simulink model "BloquesP1"  (R2024a)
settings: Solver=VariableStepAuto  StartTime=0.0  StopTime=20  MaxStep=0.001  RelTol=1e-5
values from neighbouring files (symbols this model uses):
  Beq = 4.3    [Practica1FunOde.m]
  Bp = 0.0024    [Practica1FunOde.m]
  Fc = 0    [Practica1FunOde.m]
  g = -9.81    [Practica1FunOde.m]
  Ip = 0.0079    [Practica1FunOde.m]
  lp = 0.3302    [Practica1FunOde.m]
  Mc = 0.7031    [Practica1FunOde.m]
  Mp = 0.23    [Practica1FunOde.m]
settings Model: Creator=52331  LastModifiedBy=52331

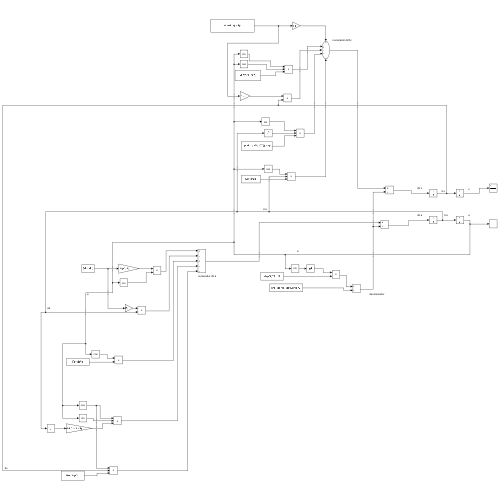
[thumbnail: Simulink's stored preview of the top-level diagram]
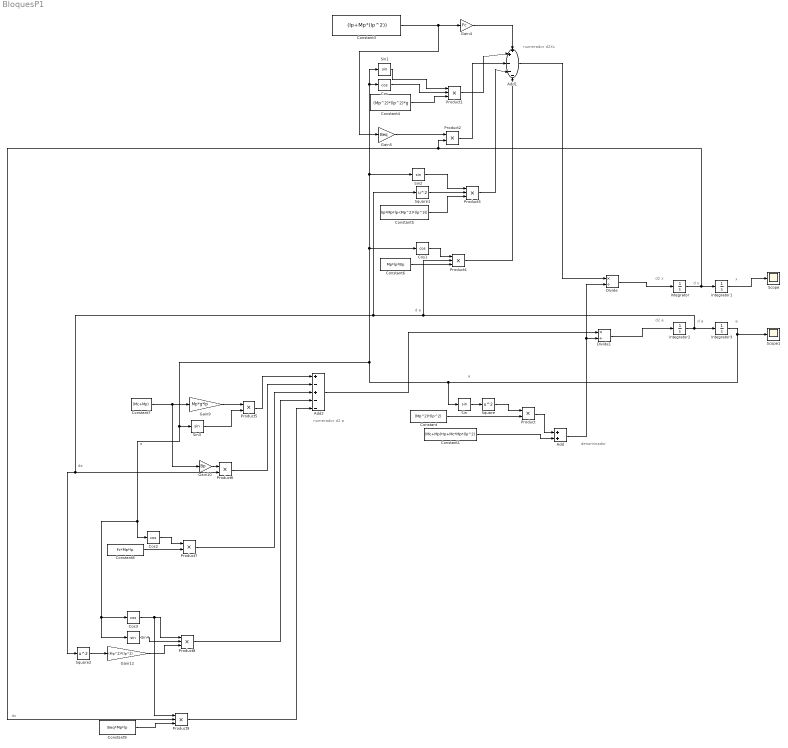
== system BloquesP1 ==
  note: numerador d2 a
  note: dx
  note: denominador
  note: numerador d2Xc
  note: a
  note: x
  note: d2 x
  note: d x
  note: d2 a
  note: a
  note: d a
  note: d a
  note: a
  note: da
  Add : Sum
  Add1 : Sum  Inputs=++---
  Add2 : Sum  Inputs=+-+--
  Constant : Constant  Value=(Mp^2)*(lp^2)
  Constant1 : Constant  Value=(Mc+Mp)*Ip+Mc*Mp*(lp^2)
  Constant3 : Constant  Value=(Ip+Mp*(lp^2))
  Constant4 : Constant  Value=(Mp^2)*(lp^2)*g
  Constant5 : Constant  Value=(Ip*Mp*lp-(Mp^2)*(lp^3))
  Constant6 : Constant  Value=Mp*lp*Bp
  Constant7 : Constant  Value=(Mc+Mp)
  Constant8 : Constant  Value=Fc*Mp*lp
  Constant9 : Constant  Value=Beq*Mp*lp
  Cos{,1..3} (4 alike) : Trigonometry  Operator=cos
  Divide : Product  Inputs=*/
  Divide1 : Product  Inputs=*/
  Gain10 : Gain  Gain=Bp
  Gain12 : Gain  Gain=(Mp^2)*(lp^2)
  Gain4 : Gain  Gain=Fc
  Gain5 : Gain  Gain=Beq
  Gain9 : Gain  Gain=Mp*g*lp
  Integrator : Integrator
  Integrator1 : Integrator
  Integrator2 : Integrator
  Integrator3 : Integrator  InitialCondition=deg2rad(1)
  Product{,2,5..7} (5 alike) : Product
  Product{1,3..4,8..9} (5 alike) : Product  Inputs=3
  Scope : Scope
  Scope1 : Scope
  Sin{,1..4} (5 alike) : Trigonometry
  Square : Math  Operator=square
  Square1 : Math  Operator=square
  Square2 : Math  Operator=square
  wires:
  Integrator/1 -> Product9/2, Product2/2, Integrator1/1
  Integrator2/1 -> Integrator3/1, Product4/2, Product6/2, Square2/1, Square1/1
  Constant1/1 -> Add/2
  Constant/1 -> Product/2
  Sin/1 -> Square/1
  Integrator3/1 -> Scope1/1, Sin4/1, Cos3/1, Cos2/1, Sin3/1, Sin1/1, Cos/1, Sin2/1, Cos1/1, Sin/1
  Product/1 -> Add/1
  Constant4/1 -> Product1/3
  Cos/1 -> Product1/2
  Sin1/1 -> Product1/1
  Product1/1 -> Add1/2
  Constant3/1 -> Gain5/1, Gain4/1
  Gain4/1 -> Add1/1
  Gain5/1 -> Product2/1
  Product2/1 -> Add1/3
  Constant5/1 -> Product3/3
  Square1/1 -> Product3/2
  Sin2/1 -> Product3/1
  Product3/1 -> Add1/4
  Constant6/1 -> Product4/3
  Cos1/1 -> Product4/1
  Product4/1 -> Add1/5
  Add1/1 -> Divide/1
  Add/1 -> Divide1/2, Divide/2
  Divide/1 -> Integrator/1
  Constant7/1 -> Gain10/1, Gain9/1
  Gain9/1 -> Product5/1
  Sin3/1 -> Product5/2
  Product5/1 -> Add2/1
  Gain10/1 -> Product6/1
  Product6/1 -> Add2/2
  Constant8/1 -> Product7/2
  Cos2/1 -> Product7/1
  Product7/1 -> Add2/3
  Gain12/1 -> Product8/3
  Square2/1 -> Gain12/1
  Cos3/1 -> Product9/1, Product8/1
  Sin4/1 -> Product8/2
  Product8/1 -> Add2/4
  Constant9/1 -> Product9/3
  Product9/1 -> Add2/5
  Divide1/1 -> Integrator2/1
  Add2/1 -> Divide1/1
  Integrator1/1 -> Scope/1
  Square/1 -> Product/1
